simulink model "WMMSupportingForcesGP2020a"  (R2020a)
settings: Solver=ode23t  StartTime=0.0  StopTime=inf  FixedStep=.001  RelTol=1e-3  AbsTol=1e-3
InitFcn:
  | InitializeSimulationGP
  | SimulationParametersGP
values from neighbouring files (symbols this model uses):
  B11_r_B11C = [0.23805608; 0.13201777; 0]    [InitializeSimulationGP.m]
  B11_r_B11Tc1 = [L11; 0; 0]    [InitializeSimulationGP.m]
  B11_Rot_Tc1 = eye(3)    [InitializeSimulationGP.m]
  B11cI = [0.28426000 -0.06487287 0;         -0.06487287  0.54237481 0;                   0  0          0.67891020]    [InitializeSimulationGP.m]
  B12_r_B12C = [0.60504569; 0.27199376; 0.00002484]    [InitializeSimulationGP.m]
  B12_r_B12Tc2 = [L12;0;0]    [InitializeSimulationGP.m]
  B12_Rot_Tc2 = eye(3)    [InitializeSimulationGP.m]
  B12cI = [1.18803886 -2.36786418 0.00280315;          -2.36786418 6.31493281 0.00022322;           0.00280315 0.00022322 7.40915161]    [InitializeSimulationGP.m]
  B31_r_B31C = [0.35781210 0 0]    [InitializeSimulationGP.m]
  B31_Rot_B41 = eye(3)    [InitializeSimulationGP.m]
  B31cI = diag([0.03150902 0.90735702 0.90763033])    [InitializeSimulationGP.m]
  B32_r_B32C = [0.35781210 0 0]    [InitializeSimulationGP.m]
  B32_Rot_B42 = eye(3)    [InitializeSimulationGP.m]
  B32cI = diag([0.03150902 0.90735702 0.90763033])    [InitializeSimulationGP.m]
  B41_r_B41C = [0.55785997 0 0]    [InitializeSimulationGP.m]
  B41_r_B41Tc1 = [lc1;0;0]    [InitializeSimulationGP.m]
  B41cI = diag([0.00370720 0.55759812 0.55785997])    [InitializeSimulationGP.m]
  B42_r_B42C = [0.55785997 0 0]    [InitializeSimulationGP.m]
  B42_r_B42Tc2 = [lc2; 0; 0]    [InitializeSimulationGP.m]
  B42cI = diag([0.00370720 0.55759812 0.55785997])    [InitializeSimulationGP.m]
  B52_r_B52C = [0 0 0.56802906]    [InitializeSimulationGP.m]
  B52_r_B52P32 = [lc3; 0; 0]    [InitializeSimulationGP.m]
  B52_Rot_P32 = eye(3)    [InitializeSimulationGP.m]
  B52cI = diag([0.91789884, 0.91790043, 0.00091463])    [InitializeSimulationGP.m]
  Bc1_r_Bc1B11 = [L1; 0; 0]    [InitializeSimulationGP.m]
  Bc1_r_Bc1B31 = [0;0;0]    [InitializeSimulationGP.m]
  Bc1_r_Bc1C = [0.14178771; 0.16555780; 0]    [InitializeSimulationGP.m]
  Bc1_V = [0;0;0;0;0;0]    [InitializeSimulationGP.m]
  Bc1cI = [+5.892211080 +5.476111360 -0.000019630;          +5.476111360 +28.66965601 -0.000024550;          -0.000019630 -0.000024550 +29.78955950]    [InitializeSimulationGP.m]
  Bc2_r_Bc2B12 = [L2;0;0]    [InitializeSimulationGP.m]
  Bc2_r_Bc2B32 = [0;0;0]    [InitializeSimulationGP.m]
  Bc2_r_Bc2C = [0.54319901; 0.10543875; 0]    [InitializeSimulationGP.m]
  Bc2cI = [0.48071390 0.52924041 0;          0.52924041 5.80912352 0;              0      0          5.97255351]    [InitializeSimulationGP.m]
  BC_r_BCBM = [xCA; yCA; zCA]    [SimulationParametersGP.m]
  BC_Rot_BM = eye(3)    [SimulationParametersGP.m]
  BCI = diag([100 1200 1000])    [SimulationParametersGP.m]
  beta1 = atan2d(374.261,935)*pi/180    [InitializeSimulationGP.m]
  beta2 = atan2d(45.757,373.313)*pi/180    [InitializeSimulationGP.m]
  beta3 = atan2d(139.50,1132.19)*pi/180    [InitializeSimulationGP.m]
  beta4 = atan2d(88.061,296.198)*pi/180    [InitializeSimulationGP.m]
  betaGround = 1e6    (= 1000000)    [SimulationParametersGP.m]
  BFL = 0.05    [SimulationParametersGP.m]
  BFR = 0.05    [SimulationParametersGP.m]
  BM_r_BMBMp = [0;0;0]    [SimulationParametersGP.m]
  BM_Rot_BMp = [cos(gamma) -sin(gamma) 0; sin(gamma) cos(gamma) 0; 0 0 1]    [SimulationParametersGP.m]
  BMp_r_BMpBc1 = [0.185;0;0.205]    [InitializeSimulationGP.m]
  BMp_Rot_Bc1 = [cos(alpha1) -sin(alpha1)  0;                  0            0       -1;                sin(alpha1)  cos(alpha1)  0]    [InitializeSimulationGP.m]
  BRL = 0.05    [SimulationParametersGP.m]
  BRR = 0.05    [SimulationParametersGP.m]
  cc = 0.0    (= 0)    [SimulationParametersGP.m]
  D22F = [0;0;0;0;0;0]    [InitializeSimulationGP.m]
  dT = 0.01    [SimulationParametersGP.m]
  g0 = 9.8066    [SimulationParametersGP.m]
  ground_stiffness = 1e8    (= 100000000)    [SimulationParametersGP.m]
  l1 = 1.15-cc    (= 1.15)    [SimulationParametersGP.m]
  L1 = 1.0071227324212    (= 1.00712273242)    [InitializeSimulationGP.m]
  L11 = 0.37610632101293    (= 0.376106321013)    [InitializeSimulationGP.m]
  L12 = 0.30901132665325    (= 0.309011326653)    [InitializeSimulationGP.m]
  l2 = 1.15+cc    (= 1.15)    [SimulationParametersGP.m]
  L2 = 1.132185817991    (= 1.13218581799)    [InitializeSimulationGP.m]
  lc1 = 0.745    [InitializeSimulationGP.m]
  lc2 = 0.745    [InitializeSimulationGP.m]
  mB11 = 25.52660174    [InitializeSimulationGP.m]
  mB12 = 33.92850233    [InitializeSimulationGP.m]
  mB31 = 17.36281648    [InitializeSimulationGP.m]
  mB32 = 17.36281648    [InitializeSimulationGP.m]
  mB41 = 10.34519231    [InitializeSimulationGP.m]
  mB42 = 10.34519231    [InitializeSimulationGP.m]
  mB52 = 6.73059863    [InitializeSimulationGP.m]
  mBC = 2200    [SimulationParametersGP.m]
  mBc1 = 307.29601379    [InitializeSimulationGP.m]
  mBc2 = 54.58702836    [InitializeSimulationGP.m]
  mFL = 60    [SimulationParametersGP.m]
  mFR = 60    [SimulationParametersGP.m]
  mP22 = 9.26136143    [InitializeSimulationGP.m]
  mP32 = 570.18877059    [InitializeSimulationGP.m]
  mRR = 60    [SimulationParametersGP.m]
  mw = mFL    (= 60)    [SimulationParametersGP.m]
  P22_r_P22C = [0.62192523 0 0]    [InitializeSimulationGP.m]
  P22_Rot_B52 = eye(3)    [InitializeSimulationGP.m]
  P22cI = diag([0.00662754, 1.48387017, 1.48398069])    [InitializeSimulationGP.m]
  P32_r_P32C = [0.25466704; -0.13034397; -0.01302248]    [InitializeSimulationGP.m]
  P32_r_P32D22 = [0.40499744871392; -0.13130517281345; -0.013385243295654]    [InitializeSimulationGP.m]
  P32_Rot_D22 = [1 0 0;              0 0.9707729441837 0.23999977258512;              0 -0.23999977258512 0.9707729441837]    [InitializeSimulationGP.m]
  P32cI = [46.81220713 0.38607676 -0.00453819;          0.38607676 71.92201786 -1.14320993;          -0.00453819 -1.14320993 67.38128576]    [InitializeSimulationGP.m]
  R0FL = 0.35    [SimulationParametersGP.m]
  R0FR = 0.35    [SimulationParametersGP.m]
  R0RL = 0.35    [SimulationParametersGP.m]
  R0RR = 0.35    [SimulationParametersGP.m]
  Rw = R0FL    (= 0.35)    [SimulationParametersGP.m]
  Tc1_r_Tc1Bc2 = [0.098495302558553; 0.01838181329939; 0]    [InitializeSimulationGP.m]
  Tc1_Rot_Bc2 = [cos(alpha2) -sin(alpha2) 0;                sin(alpha2)  cos(alpha2) 0;                0            0           1]    [InitializeSimulationGP.m]
  Tc2_r_Tc2P22 = [-0.048858374920227;0.36587359346146;0.035276938723102]    [InitializeSimulationGP.m]
  Tc2_Rot_P22 = [0.95853460763586 -0.27664713597974  0.0683942111482;                0.28497614981675  0.93051946315663 -0.23004808784757;                0                 0.23999977258511  0.9707729441837]    [InitializeSimulationGP.m]
  Th1A = 10*pi/180    (= 0.174532925199)    [InitializeSimulationGP.m]
  Th1B = 20*pi/180    (= 0.349065850399)    [InitializeSimulationGP.m]
  Th1f = 1    [InitializeSimulationGP.m]
  Th2A = 15*pi/180    (= 0.261799387799)    [InitializeSimulationGP.m]
  Th2B = -70*pi/180    (= -1.2217304764)    [InitializeSimulationGP.m]
  Th2f = 2    [InitializeSimulationGP.m]
  w = wFL    (= 0.875)    [SimulationParametersGP.m]
  W_r_WBc1 = [0.185;0;0.205]    [InitializeSimulationGP.m]
  W_Rot_Bc1 = [cos(alpha1) -sin(alpha1)  0;                  0            0       -1;                sin(alpha1)  cos(alpha1)  0]    [InitializeSimulationGP.m]
  x10 = 0.83    [InitializeSimulationGP.m]
  x20 = 0.83    [InitializeSimulationGP.m]
  x3A = 0.2    [InitializeSimulationGP.m]
  x3B = 0.3    [InitializeSimulationGP.m]
  x3f = 1    [InitializeSimulationGP.m]
  xCA = 0.5    [SimulationParametersGP.m]
  xf = [1;0;0;0;0;0]    [InitializeSimulationGP.m]
  yCA = 0    [SimulationParametersGP.m]
  zC = 0.45    [SimulationParametersGP.m]
  zCA = .25    (= 0.25)    [SimulationParametersGP.m]
  ztau = [0;0;0;0;0;1]    [InitializeSimulationGP.m]
undefined symbols (not defined in the file or in its folder): alphaFL_meas, alphaFR_meas, alphaRL_meas, alphaRR_meas, B11_V, B11Ftot, B12_U_Tc2, B12_V, B12Ftot, B31_r_B31B41, B31_V, B31FTot, B32_r_B32B42, B32_U_B42, B32_V, B32FTot, B41_V, B41FTot, B42_Rot_Tc2, B42_U_Tc2, B42_V, B42FTot, B52_U_P32, B52_V, B52Ftot, Bc1Tot, Bc2_Rot_B12, Bc2_Rot_B32, Bc2_U_B12, Bc2_U_B32, Bc2_V, Bc2Tot, betaC_meas, D22_V, deltaFL_cmd, deltaFL_meas, deltaFR_cmd, deltaFR_meas, deltaRL_cmd, deltaRL_meas, deltaRR_cmd, deltaRR_meas, dOmegaFL_meas, dOmegaFR_meas, dOmegaRL_meas, dOmegaRR_meas, dPsi_meas, dq1, dq11, dq12, dq2, dq21, dq22, dx1, dx2, Floor, FTot_S1, FTot_S2P, FTot_S2R, FzFL ... (+63)
libraries: sm_lib x94, nesl_utility x63, simulink x5
(part 5 of 11)

== system WMMSupportingForcesGP2020a/Mobile Manipulator in Simscape/get_measurements ==
  MATLAB Function : MATLAB Function  TreatAsAtomicUnit=on
  PS-Simulink Converter{1..2,15..16} (4 alike) : nesl_utility/PS-Simulink Converter  PhysicalDomain=network_engine_domain  SubClassName=ps_output  LeftPortType=input  RightPortType=output  PseudoPeriodic=off  Frequencies=[]  Unit=inherit  AffineConversion=off
      settings: SourceProductBaseCode=PW,SS
  Rate Transition{,1..5} (6 alike) : RateTransition  OutPortSampleTime=dT
  Reshape : Reshape  OutputDimensionality=Customize  OutputDimensions=[3,3]
  measVCwrtW : sm_lib/Frames and Transforms/Transform Sensor  MeasurementFrame=NonRotatingFollower  SenseAngle=off  SenseAxis=off  SenseAngle1=off  SenseAngle2=off  SenseAngle3=off  SenseQ=off  SenseR=on  SenseOmegaX=off  SenseOmegaY=off  SenseOmegaZ=on  SenseOmega1=off  SenseOmega2=off  SenseOmega3=off  SenseQDot=off  SenseRDot=off  SenseAlphaX=off  SenseAlphaY=off  SenseAlphaZ=off  SenseAlpha1=off  SenseAlpha2=off  SenseAlpha3=off  SenseQDDot=off  SenseRDDot=off  SenseX=off  SenseY=off  SenseZ=off  SenseRad=off  SenseAzim=off  SenseDist=off  SenseInc=off  SenseXDot=on  SenseYDot=on  SenseZDot=off  SenseRadDot=off  SenseAzimDot=off  SenseDistDot=off  SenseIncDot=off  SenseXDDot=off  SenseYDDot=off  SenseZDDot=off  SenseRadDDot=off  SenseAzimDDot=off  SenseDistDDot=off  SenseIncDDot=off
  W : PMIOPort  Side=Left
  BC : PMIOPort  Port=2  Side=Left
  Theta_meas : Outport
  Phi_meas : Outport  Port=2
  Psi_meas : Outport  Port=3
  dPsi_meas : Outport  Port=4
  VCx_meas : Outport  Port=5
  VCy_meas : Outport  Port=6
  wires:
  PS-Simulink Converter15/1 -> Rate Transition/1
  PS-Simulink Converter1/1 -> Reshape/1
  Reshape/1 -> MATLAB Function/1(u)
  Rate Transition/1 -> dPsi_meas/1
  PS-Simulink Converter16/1 -> Rate Transition1/1
  Rate Transition1/1 -> VCx_meas/1
  PS-Simulink Converter2/1 -> Rate Transition2/1
  Rate Transition2/1 -> VCy_meas/1
  MATLAB Function/3(Psi) -> Rate Transition4/1
  MATLAB Function/2(Phi) -> Rate Transition3/1
  MATLAB Function/1(Theta) -> Rate Transition5/1
  Rate Transition4/1 -> Psi_meas/1
  Rate Transition3/1 -> Phi_meas/1
  Rate Transition5/1 -> Theta_meas/1
  connections:
  BC/RConn1 -- measVCwrtW/RConn1
  W/RConn1 -- measVCwrtW/LConn1
  measVCwrtW/RConn2 -- PS-Simulink Converter1/LConn1
  measVCwrtW/RConn5 -- PS-Simulink Converter2/LConn1
  measVCwrtW/RConn3 -- PS-Simulink Converter15/LConn1
  measVCwrtW/RConn4 -- PS-Simulink Converter16/LConn1

== system WMMSupportingForcesGP2020a/Mobile Manipulator in Simscape/meas_FLwheel_kinematic_quantities_in_Simscape ==
  Bus Creator : BusCreator  Inputs=alphaFL_meas,VFL_meas,VxFL_meas,dOmegaFL_meas,kappaFL_meas,ReFL
  Connection Label1 : ConnectionLabel  Label=W
  Connection Label2 : ConnectionLabel  Label=W
  Connection Label56 : ConnectionLabel  Label=W
  Constant : Constant  Value=R0FL
  PS-Simulink Converter1 : nesl_utility/PS-Simulink Converter  PhysicalDomain=network_engine_domain  SubClassName=ps_output  LeftPortType=input  RightPortType=output  PseudoPeriodic=off  Frequencies=[]  Unit=inherit  AffineConversion=off
      settings: SourceProductBaseCode=PW,SS
  PS-Simulink Converter2 : nesl_utility/PS-Simulink Converter  PhysicalDomain=network_engine_domain  SubClassName=ps_output  LeftPortType=input  RightPortType=output  PseudoPeriodic=off  Frequencies=[]  Unit=inherit  AffineConversion=off
      settings: SourceProductBaseCode=PW,SS
  PS-Simulink Converter4 : nesl_utility/PS-Simulink Converter  PhysicalDomain=network_engine_domain  SubClassName=ps_output  LeftPortType=input  RightPortType=output  PseudoPeriodic=off  Frequencies=[]  Unit=inherit  AffineConversion=off
      settings: SourceProductBaseCode=PW,SS
  calc_longitudinal_slip_FL : Subsystem
  meas_VFL : Subsystem
  meas_VFL1 : Subsystem
  meas_WFL_to_W_in_WFL : sm_lib/Frames and Transforms/Transform Sensor  MeasurementFrame=NonRotatingFollower  SenseAngle=off  SenseAxis=off  SenseAngle1=off  SenseAngle2=off  SenseAngle3=off  SenseQ=off  SenseR=off  SenseOmegaX=off  SenseOmegaY=off  SenseOmegaZ=off  SenseOmega1=off  SenseOmega2=off  SenseOmega3=off  SenseQDot=off  SenseRDot=off  SenseAlphaX=off  SenseAlphaY=off  SenseAlphaZ=off  SenseAlpha1=off  SenseAlpha2=off  SenseAlpha3=off  SenseQDDot=off  SenseRDDot=off  SenseX=off  SenseY=off  SenseZ=off  SenseRad=off  SenseAzim=off  SenseDist=off  SenseInc=off  SenseXDot=on  SenseYDot=on  SenseZDot=off  SenseRadDot=off  SenseAzimDot=off  SenseDistDot=off  SenseIncDot=off  SenseXDDot=off  SenseYDDot=off  SenseZDDot=off  SenseRadDDot=off  SenseAzimDDot=off  SenseDistDDot=off  SenseIncDDot=off
  meas_WFLp_to_W_in_WFLp : sm_lib/Frames and Transforms/Transform Sensor  MeasurementFrame=NonRotatingFollower  SenseAngle=off  SenseAxis=off  SenseAngle1=off  SenseAngle2=off  SenseAngle3=off  SenseQ=off  SenseR=off  SenseOmegaX=off  SenseOmegaY=on  SenseOmegaZ=off  SenseOmega1=off  SenseOmega2=off  SenseOmega3=off  SenseQDot=off  SenseRDot=off  SenseAlphaX=off  SenseAlphaY=off  SenseAlphaZ=off  SenseAlpha1=off  SenseAlpha2=off  SenseAlpha3=off  SenseQDDot=off  SenseRDDot=off  SenseX=off  SenseY=off  SenseZ=off  SenseRad=off  SenseAzim=off  SenseDist=off  SenseInc=off  SenseXDot=off  SenseYDot=off  SenseZDot=off  SenseRadDot=off  SenseAzimDot=off  SenseDistDot=off  SenseIncDot=off  SenseXDDot=off  SenseYDDot=off  SenseZDDot=off  SenseRadDDot=off  SenseAzimDDot=off  SenseDistDDot=off  SenseIncDDot=off
  W : PMIOPort  Side=Left
  WFL : PMIOPort  Port=2  Side=Left
  WFLp : PMIOPort  Port=3  Side=Left
  FL_kin : Outport
  wires:
  [kappaFL_meas] -> Bus Creator/5  "kappaFL_meas"
  [dOmegaFL_meas] -> Bus Creator/4  "dOmegaFL_meas"
  [VxFL_meas] -> calc_longitudinal_slip_FL/3(VxFL_meas)
  [ReFL] -> calc_longitudinal_slip_FL/2(ReFL)
  Constant/1 -> [ReFL]
  [dOmegaFL_meas] -> calc_longitudinal_slip_FL/1(dOmegaFL_meas)
  calc_longitudinal_slip_FL/1(kappaFL_meas) -> [kappaFL_meas]
  PS-Simulink Converter1/1 -> [dOmegaFL_meas]
  [VxFL_meas] -> meas_VFL/1(VFLx_meas)
  [VyFL_meas] -> meas_VFL/2(VFLy_meas)
  PS-Simulink Converter2/1 -> [VxFL_meas]
  PS-Simulink Converter4/1 -> [VyFL_meas]
  [alphaFL_meas] -> Bus Creator/1  "alphaFL_meas"
  meas_VFL/1(VFL_meas) -> [VFL_meas]
  [VFL_meas] -> Bus Creator/2  "VFL_meas"
  [VxFL_meas] -> Bus Creator/3  "VxFL_meas"
  Bus Creator/1 -> [FL_kin]
  [ReFL] -> Bus Creator/6  "ReFL"
  [FL_kin] -> FL_kin/1
  [VyFL_meas] -> meas_VFL1/2(VFLy_meas)
  [VxFL_meas] -> meas_VFL1/1(VFLx_meas)
  meas_VFL1/1(alphaFL_meas) -> [alphaFL_meas]
  connections:
  meas_WFLp_to_W_in_WFLp/RConn1 -- WFLp/RConn1
  Connection Label1/LConn1 -- meas_WFL_to_W_in_WFL/LConn1
  Connection Label56/LConn1 -- W/RConn1
  PS-Simulink Converter1/LConn1 -- meas_WFLp_to_W_in_WFLp/RConn2
  Connection Label2/LConn1 -- meas_WFLp_to_W_in_WFLp/LConn1
  meas_WFL_to_W_in_WFL/RConn3 -- PS-Simulink Converter4/LConn1
  PS-Simulink Converter2/LConn1 -- meas_WFL_to_W_in_WFL/RConn2
  meas_WFL_to_W_in_WFL/RConn1 -- WFL/RConn1

== system WMMSupportingForcesGP2020a/Mobile Manipulator in Simscape/meas_FRwheel_kinematic_quantities_in_Simscape ==
  Bus Creator : BusCreator  Inputs=alphaFR_meas,VFR_meas,VxFR_meas,dOmegaFR_meas,kappaFR_meas,ReFR
  Connection Label1 : ConnectionLabel  Label=W
  Connection Label2 : ConnectionLabel  Label=W
  Connection Label56 : ConnectionLabel  Label=W
  Constant : Constant  Value=R0FR
  PS-Simulink Converter1 : nesl_utility/PS-Simulink Converter  PhysicalDomain=network_engine_domain  SubClassName=ps_output  LeftPortType=input  RightPortType=output  PseudoPeriodic=off  Frequencies=[]  Unit=inherit  AffineConversion=off
      settings: SourceProductBaseCode=PW,SS
  PS-Simulink Converter2 : nesl_utility/PS-Simulink Converter  PhysicalDomain=network_engine_domain  SubClassName=ps_output  LeftPortType=input  RightPortType=output  PseudoPeriodic=off  Frequencies=[]  Unit=inherit  AffineConversion=off
      settings: SourceProductBaseCode=PW,SS
  PS-Simulink Converter4 : nesl_utility/PS-Simulink Converter  PhysicalDomain=network_engine_domain  SubClassName=ps_output  LeftPortType=input  RightPortType=output  PseudoPeriodic=off  Frequencies=[]  Unit=inherit  AffineConversion=off
      settings: SourceProductBaseCode=PW,SS
  calc_longitudinal_slip_FR : Subsystem
  meas_VFL1 : Subsystem
  meas_VFR : Subsystem
  meas_WFR_to_W_in_WFR : sm_lib/Frames and Transforms/Transform Sensor  MeasurementFrame=NonRotatingFollower  SenseAngle=off  SenseAxis=off  SenseAngle1=off  SenseAngle2=off  SenseAngle3=off  SenseQ=off  SenseR=off  SenseOmegaX=off  SenseOmegaY=off  SenseOmegaZ=off  SenseOmega1=off  SenseOmega2=off  SenseOmega3=off  SenseQDot=off  SenseRDot=off  SenseAlphaX=off  SenseAlphaY=off  SenseAlphaZ=off  SenseAlpha1=off  SenseAlpha2=off  SenseAlpha3=off  SenseQDDot=off  SenseRDDot=off  SenseX=off  SenseY=off  SenseZ=off  SenseRad=off  SenseAzim=off  SenseDist=off  SenseInc=off  SenseXDot=on  SenseYDot=on  SenseZDot=off  SenseRadDot=off  SenseAzimDot=off  SenseDistDot=off  SenseIncDot=off  SenseXDDot=off  SenseYDDot=off  SenseZDDot=off  SenseRadDDot=off  SenseAzimDDot=off  SenseDistDDot=off  SenseIncDDot=off
  meas_WFRp_to_W_in_WFRp : sm_lib/Frames and Transforms/Transform Sensor  MeasurementFrame=NonRotatingFollower  SenseAngle=off  SenseAxis=off  SenseAngle1=off  SenseAngle2=off  SenseAngle3=off  SenseQ=off  SenseR=off  SenseOmegaX=off  SenseOmegaY=on  SenseOmegaZ=off  SenseOmega1=off  SenseOmega2=off  SenseOmega3=off  SenseQDot=off  SenseRDot=off  SenseAlphaX=off  SenseAlphaY=off  SenseAlphaZ=off  SenseAlpha1=off  SenseAlpha2=off  SenseAlpha3=off  SenseQDDot=off  SenseRDDot=off  SenseX=off  SenseY=off  SenseZ=off  SenseRad=off  SenseAzim=off  SenseDist=off  SenseInc=off  SenseXDot=off  SenseYDot=off  SenseZDot=off  SenseRadDot=off  SenseAzimDot=off  SenseDistDot=off  SenseIncDot=off  SenseXDDot=off  SenseYDDot=off  SenseZDDot=off  SenseRadDDot=off  SenseAzimDDot=off  SenseDistDDot=off  SenseIncDDot=off
  W : PMIOPort  Side=Left
  WFR : PMIOPort  Port=2  Side=Left
  WFRp : PMIOPort  Port=3  Side=Left
  FR_kin : Outport
  wires:
  meas_VFR/1(VFR_meas) -> [VFR_meas]
  PS-Simulink Converter4/1 -> [VyFR_meas]
  PS-Simulink Converter2/1 -> [VxFR_meas]
  [VyFR_meas] -> meas_VFR/2(VFRy_meas)
  [VxFR_meas] -> meas_VFR/1(VFRx_meas)
  PS-Simulink Converter1/1 -> [dOmegaFR_meas]
  calc_longitudinal_slip_FR/1(kappaFR_meas) -> [kappaFR_meas]
  [dOmegaFR_meas] -> calc_longitudinal_slip_FR/1(dOmegaFR_meas)
  Constant/1 -> [ReFR]
  [ReFR] -> calc_longitudinal_slip_FR/2(ReFR)
  [VxFR_meas] -> calc_longitudinal_slip_FR/3(VxFR_meas)
  [dOmegaFR_meas] -> Bus Creator/4  "dOmegaFR_meas"
  [VxFR_meas] -> Bus Creator/3  "VxFR_meas"
  [alphaFR_meas] -> Bus Creator/1  "alphaFR_meas"
  [VFR_meas] -> Bus Creator/2  "VFR_meas"
  [kappaFR_meas] -> Bus Creator/5  "kappaFR_meas"
  Bus Creator/1 -> [FR_kin]
  [FR_kin] -> FR_kin/1
  [ReFR] -> Bus Creator/6  "ReFR"
  [VxFR_meas] -> meas_VFL1/1(VFRx_meas)
  [VyFR_meas] -> meas_VFL1/2(VFRy_meas)
  meas_VFL1/1(alphaFR_meas) -> [alphaFR_meas]
  connections:
  meas_WFR_to_W_in_WFR/RConn1 -- WFR/RConn1
  PS-Simulink Converter2/LConn1 -- meas_WFR_to_W_in_WFR/RConn2
  meas_WFR_to_W_in_WFR/RConn3 -- PS-Simulink Converter4/LConn1
  Connection Label2/LConn1 -- meas_WFRp_to_W_in_WFRp/LConn1
  PS-Simulink Converter1/LConn1 -- meas_WFRp_to_W_in_WFRp/RConn2
  Connection Label56/LConn1 -- W/RConn1
  Connection Label1/LConn1 -- meas_WFR_to_W_in_WFR/LConn1
  meas_WFRp_to_W_in_WFRp/RConn1 -- WFRp/RConn1

== system WMMSupportingForcesGP2020a/Mobile Manipulator in Simscape/meas_RLwheel_kinematic_quantities_in_Simscape ==
  Bus Creator : BusCreator  Inputs=alphaRL_meas,VRL_meas,VxRL_meas,dOmegaRL_meas,kappaRL_meas,ReRL
  Connection Label1 : ConnectionLabel  Label=W
  Connection Label2 : ConnectionLabel  Label=W
  Connection Label56 : ConnectionLabel  Label=W
  Constant : Constant  Value=R0RL
  PS-Simulink Converter1 : nesl_utility/PS-Simulink Converter  PhysicalDomain=network_engine_domain  SubClassName=ps_output  LeftPortType=input  RightPortType=output  PseudoPeriodic=off  Frequencies=[]  Unit=inherit  AffineConversion=off
      settings: SourceProductBaseCode=PW,SS
  PS-Simulink Converter2 : nesl_utility/PS-Simulink Converter  PhysicalDomain=network_engine_domain  SubClassName=ps_output  LeftPortType=input  RightPortType=output  PseudoPeriodic=off  Frequencies=[]  Unit=inherit  AffineConversion=off
      settings: SourceProductBaseCode=PW,SS
  PS-Simulink Converter4 : nesl_utility/PS-Simulink Converter  PhysicalDomain=network_engine_domain  SubClassName=ps_output  LeftPortType=input  RightPortType=output  PseudoPeriodic=off  Frequencies=[]  Unit=inherit  AffineConversion=off
      settings: SourceProductBaseCode=PW,SS
  calc_longitudinal_slip_RL : Subsystem
  meas_VFL1 : Subsystem
  meas_VRL : Subsystem
  meas_WRL_to_W_in_WRL : sm_lib/Frames and Transforms/Transform Sensor  MeasurementFrame=NonRotatingFollower  SenseAngle=off  SenseAxis=off  SenseAngle1=off  SenseAngle2=off  SenseAngle3=off  SenseQ=off  SenseR=off  SenseOmegaX=off  SenseOmegaY=off  SenseOmegaZ=off  SenseOmega1=off  SenseOmega2=off  SenseOmega3=off  SenseQDot=off  SenseRDot=off  SenseAlphaX=off  SenseAlphaY=off  SenseAlphaZ=off  SenseAlpha1=off  SenseAlpha2=off  SenseAlpha3=off  SenseQDDot=off  SenseRDDot=off  SenseX=off  SenseY=off  SenseZ=off  SenseRad=off  SenseAzim=off  SenseDist=off  SenseInc=off  SenseXDot=on  SenseYDot=on  SenseZDot=off  SenseRadDot=off  SenseAzimDot=off  SenseDistDot=off  SenseIncDot=off  SenseXDDot=off  SenseYDDot=off  SenseZDDot=off  SenseRadDDot=off  SenseAzimDDot=off  SenseDistDDot=off  SenseIncDDot=off
  meas_WRLp_to_W_in_WRLp : sm_lib/Frames and Transforms/Transform Sensor  MeasurementFrame=NonRotatingFollower  SenseAngle=off  SenseAxis=off  SenseAngle1=off  SenseAngle2=off  SenseAngle3=off  SenseQ=off  SenseR=off  SenseOmegaX=off  SenseOmegaY=on  SenseOmegaZ=off  SenseOmega1=off  SenseOmega2=off  SenseOmega3=off  SenseQDot=off  SenseRDot=off  SenseAlphaX=off  SenseAlphaY=off  SenseAlphaZ=off  SenseAlpha1=off  SenseAlpha2=off  SenseAlpha3=off  SenseQDDot=off  SenseRDDot=off  SenseX=off  SenseY=off  SenseZ=off  SenseRad=off  SenseAzim=off  SenseDist=off  SenseInc=off  SenseXDot=off  SenseYDot=off  SenseZDot=off  SenseRadDot=off  SenseAzimDot=off  SenseDistDot=off  SenseIncDot=off  SenseXDDot=off  SenseYDDot=off  SenseZDDot=off  SenseRadDDot=off  SenseAzimDDot=off  SenseDistDDot=off  SenseIncDDot=off
  W : PMIOPort  Side=Left
  WRL : PMIOPort  Port=2  Side=Left
  WRLp : PMIOPort  Port=3  Side=Left
  RL_kin : Outport
  wires:
  meas_VRL/1(VRL_meas) -> [VRL_meas]
  PS-Simulink Converter4/1 -> [VyRL_meas]
  PS-Simulink Converter2/1 -> [VxRL_meas]
  [VyRL_meas] -> meas_VRL/2(VRLy_meas)
  [VxRL_meas] -> meas_VRL/1(VRLx_meas)
  PS-Simulink Converter1/1 -> [dOmegaRL_meas]
  calc_longitudinal_slip_RL/1(kappaRL_meas) -> [kappaRL_meas]
  [dOmegaRL_meas] -> calc_longitudinal_slip_RL/1(dOmegaRL_meas)
  Constant/1 -> [ReRL]
  [ReRL] -> calc_longitudinal_slip_RL/2(ReRL)
  [VxRL_meas] -> calc_longitudinal_slip_RL/3(VxRL_meas)
  [dOmegaRL_meas] -> Bus Creator/4  "dOmegaRL_meas"
  [VxRL_meas] -> Bus Creator/3  "VxRL_meas"
  [alphaRL_meas] -> Bus Creator/1  "alphaRL_meas"
  [VRL_meas] -> Bus Creator/2  "VRL_meas"
  [kappaRL_meas] -> Bus Creator/5  "kappaRL_meas"
  Bus Creator/1 -> [RL_kin]
  [RL_kin] -> RL_kin/1
  [ReRL] -> Bus Creator/6  "ReRL"
  [VxRL_meas] -> meas_VFL1/1(VRLx_meas)
  [VyRL_meas] -> meas_VFL1/2(VRLy_meas)
  meas_VFL1/1(alphaRL_meas) -> [alphaRL_meas]
  connections:
  meas_WRL_to_W_in_WRL/RConn1 -- WRL/RConn1
  PS-Simulink Converter2/LConn1 -- meas_WRL_to_W_in_WRL/RConn2
  meas_WRL_to_W_in_WRL/RConn3 -- PS-Simulink Converter4/LConn1
  Connection Label2/LConn1 -- meas_WRLp_to_W_in_WRLp/LConn1
  PS-Simulink Converter1/LConn1 -- meas_WRLp_to_W_in_WRLp/RConn2
  Connection Label56/LConn1 -- W/RConn1
  Connection Label1/LConn1 -- meas_WRL_to_W_in_WRL/LConn1
  meas_WRLp_to_W_in_WRLp/RConn1 -- WRLp/RConn1

== system WMMSupportingForcesGP2020a/Mobile Manipulator in Simscape/meas_RRwheel_kinematic_quantities_in_Simscape ==
  Bus Creator : BusCreator  Inputs=alphaRR_meas,VRR_meas,VxRR_meas,dOmegaRR_meas,kappaRR_meas,ReRR
  Connection Label1 : ConnectionLabel  Label=W
  Connection Label2 : ConnectionLabel  Label=W
  Connection Label56 : ConnectionLabel  Label=W
  Constant : Constant  Value=R0RR
  PS-Simulink Converter1 : nesl_utility/PS-Simulink Converter  PhysicalDomain=network_engine_domain  SubClassName=ps_output  LeftPortType=input  RightPortType=output  PseudoPeriodic=off  Frequencies=[]  Unit=inherit  AffineConversion=off
      settings: SourceProductBaseCode=PW,SS
  PS-Simulink Converter2 : nesl_utility/PS-Simulink Converter  PhysicalDomain=network_engine_domain  SubClassName=ps_output  LeftPortType=input  RightPortType=output  PseudoPeriodic=off  Frequencies=[]  Unit=inherit  AffineConversion=off
      settings: SourceProductBaseCode=PW,SS
  PS-Simulink Converter4 : nesl_utility/PS-Simulink Converter  PhysicalDomain=network_engine_domain  SubClassName=ps_output  LeftPortType=input  RightPortType=output  PseudoPeriodic=off  Frequencies=[]  Unit=inherit  AffineConversion=off
      settings: SourceProductBaseCode=PW,SS
  calc_longitudinal_slip_RR : Subsystem
  meas_VFL1 : Subsystem
  meas_VRR : Subsystem
  meas_WRR_to_W_in_WRR : sm_lib/Frames and Transforms/Transform Sensor  MeasurementFrame=NonRotatingFollower  SenseAngle=off  SenseAxis=off  SenseAngle1=off  SenseAngle2=off  SenseAngle3=off  SenseQ=off  SenseR=off  SenseOmegaX=off  SenseOmegaY=off  SenseOmegaZ=off  SenseOmega1=off  SenseOmega2=off  SenseOmega3=off  SenseQDot=off  SenseRDot=off  SenseAlphaX=off  SenseAlphaY=off  SenseAlphaZ=off  SenseAlpha1=off  SenseAlpha2=off  SenseAlpha3=off  SenseQDDot=off  SenseRDDot=off  SenseX=off  SenseY=off  SenseZ=off  SenseRad=off  SenseAzim=off  SenseDist=off  SenseInc=off  SenseXDot=on  SenseYDot=on  SenseZDot=off  SenseRadDot=off  SenseAzimDot=off  SenseDistDot=off  SenseIncDot=off  SenseXDDot=off  SenseYDDot=off  SenseZDDot=off  SenseRadDDot=off  SenseAzimDDot=off  SenseDistDDot=off  SenseIncDDot=off
  meas_WRRp_to_W_in_WRRp : sm_lib/Frames and Transforms/Transform Sensor  MeasurementFrame=NonRotatingFollower  SenseAngle=off  SenseAxis=off  SenseAngle1=off  SenseAngle2=off  SenseAngle3=off  SenseQ=off  SenseR=off  SenseOmegaX=off  SenseOmegaY=on  SenseOmegaZ=off  SenseOmega1=off  SenseOmega2=off  SenseOmega3=off  SenseQDot=off  SenseRDot=off  SenseAlphaX=off  SenseAlphaY=off  SenseAlphaZ=off  SenseAlpha1=off  SenseAlpha2=off  SenseAlpha3=off  SenseQDDot=off  SenseRDDot=off  SenseX=off  SenseY=off  SenseZ=off  SenseRad=off  SenseAzim=off  SenseDist=off  SenseInc=off  SenseXDot=off  SenseYDot=off  SenseZDot=off  SenseRadDot=off  SenseAzimDot=off  SenseDistDot=off  SenseIncDot=off  SenseXDDot=off  SenseYDDot=off  SenseZDDot=off  SenseRadDDot=off  SenseAzimDDot=off  SenseDistDDot=off  SenseIncDDot=off
  W : PMIOPort  Side=Left
  WRR : PMIOPort  Port=2  Side=Left
  WRRp : PMIOPort  Port=3  Side=Left
  RR_kin : Outport
  wires:
  [VxRR_meas] -> calc_longitudinal_slip_RR/3(VxRR_meas)
  [ReRR] -> calc_longitudinal_slip_RR/2(ReRR)
  Constant/1 -> [ReRR]
  [dOmegaRR_meas] -> calc_longitudinal_slip_RR/1(dOmegaRR_meas)
  calc_longitudinal_slip_RR/1(kappaRR_meas) -> [kappaRR_meas]
  PS-Simulink Converter1/1 -> [dOmegaRR_meas]
  [VxRR_meas] -> meas_VRR/1(VRRx_meas)
  [VyRR_meas] -> meas_VRR/2(VRRy_meas)
  PS-Simulink Converter2/1 -> [VxRR_meas]
  PS-Simulink Converter4/1 -> [VyRR_meas]
  meas_VRR/1(VRR_meas) -> [VRR_meas]
  [RR_kin] -> RR_kin/1
  [kappaRR_meas] -> Bus Creator/5  "kappaRR_meas"
  [ReRR] -> Bus Creator/6  "ReRR"
  Bus Creator/1 -> [RR_kin]
  [alphaRR_meas] -> Bus Creator/1  "alphaRR_meas"
  [VRR_meas] -> Bus Creator/2  "VRR_meas"
  [dOmegaRR_meas] -> Bus Creator/4  "dOmegaRR_meas"
  [VxRR_meas] -> Bus Creator/3  "VxRR_meas"
  [VxRR_meas] -> meas_VFL1/1(VRRx_meas)
  [VyRR_meas] -> meas_VFL1/2(VRRy_meas)
  meas_VFL1/1(alphaRR_meas) -> [alphaRR_meas]
  connections:
  meas_WRRp_to_W_in_WRRp/RConn1 -- WRRp/RConn1
  Connection Label1/LConn1 -- meas_WRR_to_W_in_WRR/LConn1
  Connection Label56/LConn1 -- W/RConn1
  PS-Simulink Converter1/LConn1 -- meas_WRRp_to_W_in_WRRp/RConn2
  Connection Label2/LConn1 -- meas_WRRp_to_W_in_WRRp/LConn1
  meas_WRR_to_W_in_WRR/RConn3 -- PS-Simulink Converter4/LConn1
  PS-Simulink Converter2/LConn1 -- meas_WRR_to_W_in_WRR/RConn2
  meas_WRR_to_W_in_WRR/RConn1 -- WRR/RConn1

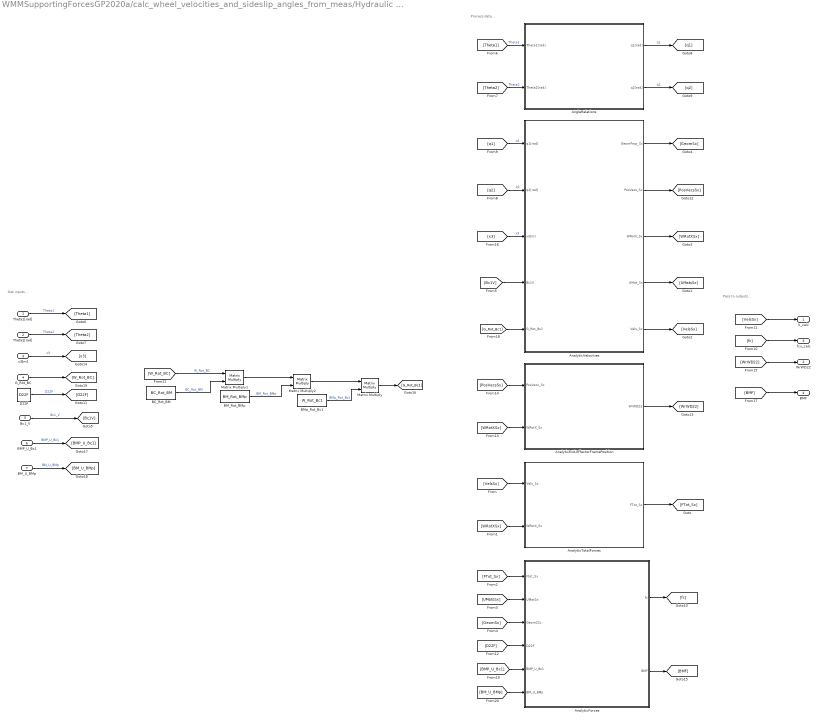
== system WMMSupportingForcesGP2020a/calc_wheel_velocities_and_sideslip_angles_from_meas/Hydraulic manipulator, calculation ==
  note: Pass to outputs...
  note: Get inputs...
  note: Process data...
  Theta1[rad] : Inport
  Theta2[rad] : Inport  Port=2
  x3[m] : Inport  Port=3
  G_Rot_BC : Inport  Port=4
  Bc1_V : Inport  Port=5
  BMP_U_Bc1 : Inport  Port=6
  BM_U_BMp : Inport  Port=7
  AnalyticEnd-EffectorFramePosition : Subsystem
  AnalyticForces : Subsystem
  AnalyticTotalForces : Subsystem
  AnalyticVelocities : Subsystem
  AngleRelations : Subsystem
  BC_Rot_BM : Constant  Value=BC_Rot_BM
  BM_Rot_BMp : Constant  Value=BM_Rot_BMp
  BMp_Rot_Bc1 : Constant  Value=W_Rot_Bc1
  D22F : Constant  Value=D22F
  Matrix Multiply : Product  Multiplication=Matrix(*)
  Matrix Multiply1 : Product  Multiplication=Matrix(*)
  Matrix Multiply2 : Product  Multiplication=Matrix(*)
  V_calc : Outport
  WrWD22 : Outport  Port=2
  fcx_calc : Outport  Port=3
  BMF : Outport  Port=4
  wires:
  AnalyticTotalForces/1(FTot_Sx) -> [FTot_Sx]
  AnalyticVelocities/1(GeomProp_Sx) -> [GeomSx]
  AnalyticVelocities/4(UMat_Sx) -> [UMatsSx]
  [UMatsSx] -> AnalyticForces/2(UMatSx)
  [VelsSx] -> AnalyticTotalForces/1(Vels_Sx)
  [GeomSx] -> AnalyticForces/3(GeomCCx)
  AnalyticVelocities/3(WRotX_Sx) -> [WRotXSx]
  [WRotXSx] -> AnalyticTotalForces/2(WRotX_Sx)
  [FTot_Sx] -> AnalyticForces/1(Ftot_Sx)
  AnalyticVelocities/5(Vels_Sx) -> [VelsSx]
  Theta1[rad]/1 -> [Theta1]  "Theta1"
  Theta2[rad]/1 -> [Theta2]  "Theta2"
  [Theta1] -> AngleRelations/1(Theta1[rad])  "Theta1"
  [Theta2] -> AngleRelations/2(Theta2[rad])  "Theta2"
  AngleRelations/1(q1[rad]) -> [q1]  "q1"
  AngleRelations/2(q2[rad]) -> [q2]  "q2"
  [q2] -> AnalyticVelocities/2(q2[rad])  "q2"
  [q1] -> AnalyticVelocities/1(q1[rad])  "q1"
  AnalyticForces/1(fc) -> [fc]
  [fc] -> fcx_calc/1
  [VelsSx] -> V_calc/1
  [D22F] -> AnalyticForces/4(D22F)
  [WRotXSx] -> AnalyticEnd-EffectorFramePosition/2(WRotX_Sx)
  AnalyticVelocities/2(PosVecs_Sx) -> [PosVecsSx]
  [PosVecsSx] -> AnalyticEnd-EffectorFramePosition/1(PosVecs_Sx)
  AnalyticEnd-EffectorFramePosition/1(WrWD22) -> [WrWD22]
  [WrWD22] -> WrWD22/1
  D22F/1 -> [D22F]  "D22F"
  x3[m]/1 -> [x3]  "x3"
  [x3] -> AnalyticVelocities/3(x3[m])  "x3"
  Bc1_V/1 -> [Bc1V]  "Bc1_V"
  [Bc1V] -> AnalyticVelocities/4(Bc1V)
  AnalyticForces/2(BMF) -> [BMF]
  [BMF] -> BMF/1
  [G_Rot_Bc1] -> AnalyticVelocities/5(G_Rot_Bc1)
  G_Rot_BC/1 -> [W_Rot_BC]
  BMP_U_Bc1/1 -> [BMP_U_Bc1]  "BMP_U_Bc1"
  [BMP_U_Bc1] -> AnalyticForces/5(BMP_U_Bc1)
  BM_U_BMp/1 -> [BM_U_BMp]  "BM_U_BMp"
  [BM_U_BMp] -> AnalyticForces/6(BM_U_BMp)
  Matrix Multiply1/1 -> Matrix Multiply2/1
  BMp_Rot_Bc1/1 -> Matrix Multiply/2  "BMp_Rot_Bc1"
  Matrix Multiply2/1 -> Matrix Multiply/1
  BC_Rot_BM/1 -> Matrix Multiply1/2  "BC_Rot_BM"
  BM_Rot_BMp/1 -> Matrix Multiply2/2  "BM_Rot_BMp"
  [W_Rot_BC] -> Matrix Multiply1/1  "W_Rot_BC"
  Matrix Multiply/1 -> [G_Rot_Bc1]

== system WMMSupportingForcesGP2020a/Mobile Manipulator in Simscape/GroundReactionFL/verticalForceFL ==
  hFL : Inport
  vzFL : Inport  Port=2
  Constant1 : Constant  Value=R0FL
  Subtract : Sum  Inputs=+-
  Sum1 : Sum  Inputs=|+-
  Tire Vertical Stiffness : Lookup_n-D  NumberOfTableDimensions=1  BreakpointsForDimension1=[-1 0 0.1]  Table=[ground_stiffness 0 0]  InternalRulePriority=Speed  RndMeth=Simplest  InputSameDT=on
  dampingForceFL : Subsystem
  FvertFL : Outport  VectorParamsAs1DForOutWhenUnconnected=off
  wires:
  Tire Vertical Stiffness/1 -> Sum1/1, dampingForceFL/1(Fz k)
  Subtract/1 -> Tire Vertical Stiffness/1
  Constant1/1 -> Subtract/2
  dampingForceFL/1(Fz d) -> Sum1/2
  vzFL/1 -> dampingForceFL/2(vz)
  Sum1/1 -> FvertFL/1
  hFL/1 -> Subtract/1

== system WMMSupportingForcesGP2020a/Mobile Manipulator in Simscape/GroundReactionFR/verticalForceFR ==
  hFR : Inport
  vzFR : Inport  Port=2
  Constant1 : Constant  Value=R0FR
  Subtract : Sum  Inputs=+-
  Sum1 : Sum  Inputs=|+-
  Tire Vertical Stiffness : Lookup_n-D  NumberOfTableDimensions=1  BreakpointsForDimension1=[-1 0 0.1]  Table=[ground_stiffness 0 0]  InternalRulePriority=Speed  RndMeth=Simplest  InputSameDT=on
  dampingForceFR : Subsystem
  FvertFR : Outport  VectorParamsAs1DForOutWhenUnconnected=off
  wires:
  Tire Vertical Stiffness/1 -> Sum1/1, dampingForceFR/1(Fz k)
  Subtract/1 -> Tire Vertical Stiffness/1
  Constant1/1 -> Subtract/2
  dampingForceFR/1(Fz d) -> Sum1/2
  vzFR/1 -> dampingForceFR/2(vz)
  Sum1/1 -> FvertFR/1
  hFR/1 -> Subtract/1

== system WMMSupportingForcesGP2020a/Mobile Manipulator in Simscape/GroundReactionRL/verticalForceRL ==
  hRL : Inport
  vzRL : Inport  Port=2
  Constant1 : Constant  Value=R0RL
  Subtract : Sum  Inputs=+-
  Sum1 : Sum  Inputs=|+-
  Tire Vertical Stiffness : Lookup_n-D  NumberOfTableDimensions=1  BreakpointsForDimension1=[-1 0 0.1]  Table=[ground_stiffness 0 0]  InternalRulePriority=Speed  RndMeth=Simplest  InputSameDT=on
  dampingForceRL : Subsystem
  FvertRL : Outport  VectorParamsAs1DForOutWhenUnconnected=off
  wires:
  Tire Vertical Stiffness/1 -> Sum1/1, dampingForceRL/1(Fz k)
  Subtract/1 -> Tire Vertical Stiffness/1
  Constant1/1 -> Subtract/2
  dampingForceRL/1(Fz d) -> Sum1/2
  vzRL/1 -> dampingForceRL/2(vz)
  Sum1/1 -> FvertRL/1
  hRL/1 -> Subtract/1

== system WMMSupportingForcesGP2020a/Mobile Manipulator in Simscape/GroundReactionRR/verticalForceRR ==
  hRR : Inport
  vzRR : Inport  Port=2
  Constant1 : Constant  Value=R0RR
  Subtract : Sum  Inputs=+-
  Sum1 : Sum  Inputs=|+-
  Tire Vertical Stiffness : Lookup_n-D  NumberOfTableDimensions=1  BreakpointsForDimension1=[-1 0 0.1]  Table=[ground_stiffness 0 0]  InternalRulePriority=Speed  RndMeth=Simplest  InputSameDT=on
  dampingForceRR : Subsystem
  FvertRR : Outport  VectorParamsAs1DForOutWhenUnconnected=off
  wires:
  Tire Vertical Stiffness/1 -> Sum1/1, dampingForceRR/1(Fz k)
  Subtract/1 -> Tire Vertical Stiffness/1
  Constant1/1 -> Subtract/2
  dampingForceRR/1(Fz d) -> Sum1/2
  vzRR/1 -> dampingForceRR/2(vz)
  Sum1/1 -> FvertRR/1
  hRR/1 -> Subtract/1

== system WMMSupportingForcesGP2020a/Mobile Manipulator in Simscape/Hydraulic manipulator, Simscape/Base ==
  note: Analytic derivatives
  Theta1[rad] : Inport
  BaseSolid : sm_lib/Body Elements/File Solid  ExtGeomFileName=01_BaseGP.STEP  UnitType=FromFile  ExtGeomFileUnits=m  StepReaderType=OCC  ExportConvexHullGeometry=off  InertiaType=Custom  Mass=307.29601379  MassUnits=kg  CenterOfMass=[0 -0.01488967 0.02139206]  CenterOfMassUnits=m  MomentsOfInertia=[29.78955950 5.25917100 29.30269608]  MomentsOfInertiaUnits=kg*m^2  ProductsOfInertia=[-3.89461427 -0.00003008 -0.00000910]  ProductsOfInertiaUnits=kg*m^2  BasedOnType=Density  Density=7300  DensityUnits=kg/m^3  DoExposeReferenceFrame=off  SerializedFrames=<Frames><Frame><Id>Frame1</Id><Value><Name>F2</Name><Origin><Source>GeometricFeature</Source><FeatureName>cylindrical surface 2</FeatureName></Origin><PrimaryAxis><DefinedDirection>+X</DefinedDirection><Source>ReferenceFrame</Source><SourceDirection>-Z</SourceDirection><FeatureName></FeatureName></PrimaryAxis><SecondaryAxis><DefinedDirection>+Y</DefinedDirection><Source>ReferenceFrame</Source><SourceDirection>+Y</SourceDirection><FeatureName></FeatureName></SecondaryAxis></Value></Frame><Frame><Id>Frame2</Id><Value><Name>F1</Name><Origin><Source>GeometricFeature</Source><FeatureName>cylindrical surface 1</FeatureName></Origin><PrimaryAxis><DefinedDirection>-X</DefinedDirection><Source>ReferenceFrame</Source><SourceDirection>+Z</SourceDirection><FeatureName></FeatureName></PrimaryAxis><SecondaryAxis><DefinedDirection>+Y</DefinedDirection><Source>ReferenceFrame</Source><SourceDirection>+Y</SourceDirection><FeatureName></FeatureName></SecondaryAxis></Value></Frame><Frame><Id>Frame3</Id><Value><Name>Bc1</Name><Origin><Source>GeometricFeature</Source><FeatureName>cylindrical surface 1</FeatureName></Origin><PrimaryAxis><DefinedDirection>+X</DefinedDirection><Source>GeometricFeature</Source><SourceDirection>+Z</SourceDirection><FeatureName>segment 135</FeatureName></PrimaryAxis><SecondaryAxis><DefinedDirection>+Y</DefinedDirection><Source>ReferenceFrame</Source><SourceDirection>+Z</SourceDirection><FeatureName></FeatureName></SecondaryAxis></Value></Frame><Frame><Id>Frame4</Id><Value><Name>BMp</Name><Origin><Source>GeometricFeature</Source><FeatureName>planar surface 11</FeatureName></Origin><PrimaryAxis><DefinedDirection>+X</DefinedDirection><Source>ReferenceFrame</Source><SourceDirection>-Z</SourceDirection><FeatureName></FeatureName></PrimaryAxis><SecondaryAxis><DefinedDirection>+Z</DefinedDirection><Source>ReferenceFrame</Source><SourceDirection>+Y</SourceDirection><FeatureName></FeatureName></SecondaryAxis></Value></Frame></Frames>  GraphicType=FromGeometry  MarkerShape=Sphere  MarkerSize=10  GraphicVisPropType=SimpleVisualProperties  GraphicDiffuseColor=[134 134 71]/255  GraphicSpecularColor=[0.5 0.5 0.5 1.0]  GraphicAmbientColor=[0.15 0.15 0.15 1.0]  GraphicEmissiveColor=[0.0 0.0 0.0 1.0]  GraphicShininess=75  GraphicOpacity=1.0
  Sim-PS1 : nesl_utility/Simulink-PS Converter  PhysicalDomain=network_engine_domain  SubClassName=ps_input  LeftPortType=input  RightPortType=output  PseudoPeriodic=off  Frequencies=[]  NoiseDistribution=none  NoiseParameters=[]  Unit=rad  AffineConversion=off  FilteringAndDerivatives=provide  SimscapeFilterOrder=2  InputFilterTimeConstant=0.001  UdotUserProvided=2
      settings: SourceProductBaseCode=PW,SS
  Sine Wave : Sin  Amplitude=Th1A*Th1f  Frequency=Th1f  Phase=pi/2  SampleTime=0
  Sine Wave1 : Sin  Amplitude=Th1A*Th1f*Th1f  Frequency=Th1f  Phase=pi  SampleTime=0
  Theta1-rotation : sm_lib/Joints/Revolute Joint  JointMode=Normal  SenseConstraintForce=off  SenseConstraintForceX=off  SenseConstraintForceY=off  SenseConstraintForceZ=off  SenseConstraintTorque=off  SenseConstraintTorqueX=off  SenseConstraintTorqueY=off  SenseConstraintTorqueZ=off  SenseTotalForce=off  SenseTotalForceX=off  SenseTotalForceY=off  SenseTotalForceZ=off  SenseTotalTorque=off  SenseTotalTorqueX=off  SenseTotalTorqueY=off  SenseTotalTorqueZ=off  CompositeWrenchDir=FollowerOnBase  CompositeWrenchFrame=BaseFrame  EquilibriumPosition=0  EquilibriumPositionUnits=rad  SpringStiffness=0  SpringStiffnessUnits=N*m/rad  DampingCoefficient=10  DampingCoefficientUnits=N*m/(rad/s)  TorqueActuationMode=NoTorque  MotionActuationMode=InputMotion  SensePosition=off  SenseVelocity=off  SenseAcceleration=off  SenseTorqueForce=off  SenseLowerLimitTorqueForce=off  SenseUpperLimitTorqueForce=off  LowerLimitSpecify=off  LowerLimitBound=-90  LowerLimitBoundUnits=deg  LowerLimitStiffness=1e4  LowerLimitStiffnessUnits=N*m/deg  LowerLimitDamping=10  LowerLimitDampingUnits=N*m/(deg/s)  LowerLimitTransitionRegionWidth=0.1  LowerLimitTransitionRegionWidthUnits=deg  UpperLimitSpecify=off  UpperLimitBound=90  UpperLimitBoundUnits=deg  UpperLimitStiffness=1e4  UpperLimitStiffnessUnits=N*m/deg  UpperLimitDamping=10  UpperLimitDampingUnits=N*m/(deg/s)  UpperLimitTransitionRegionWidth=0.1  UpperLimitTransitionRegionWidthUnits=deg  PositionTargetSpecify=on  PositionTargetPriority=Low  PositionTargetValue=Th1B  PositionTargetValueUnits=rad  VelocityTargetSpecify=off  VelocityTargetPriority=High  VelocityTargetValue=0  VelocityTargetValueUnits=deg/s
  BMp : PMIOPort  Side=Left
  Bc1 : PMIOPort  Port=2  Side=Left
  F1 : PMIOPort  Port=3  Side=Right
  F2_rot : PMIOPort  Port=4  Side=Right
  wires:
  Sine Wave/1 -> Sim-PS1/2
  Sine Wave1/1 -> Sim-PS1/3
  Theta1[rad]/1 -> Sim-PS1/1  "Theta1"
  connections:
  BaseSolid/RConn2 -- BMp/RConn1
  Theta1-rotation/LConn1 -- BaseSolid/LConn1
  Sim-PS1/RConn1 -- Theta1-rotation/LConn2
  F2_rot/RConn1 -- Theta1-rotation/RConn1
  F1/RConn1 -- BaseSolid/RConn1
  Bc1/RConn1 -- BaseSolid/LConn2

== system WMMSupportingForcesGP2020a/Mobile Manipulator in Simscape/Hydraulic manipulator, Simscape/EndMassObject ==
  EndObjectMass : sm_lib/Body Elements/File Solid  ExtGeomFileName=10_ObjectGP.STEP  UnitType=FromFile  ExtGeomFileUnits=m  StepReaderType=OCC  ExportConvexHullGeometry=off  InertiaType=Custom  Mass=570.18877059  MassUnits=kg  CenterOfMass=[2.16142487 0.01347152 0.06601658]  CenterOfMassUnits=m  MomentsOfInertia=[46.81220713 72.19317437 67.11012925]  MomentsOfInertiaUnits=kg*m^2  ProductsOfInertia=[0.04641137 0.08825278 0.37588204]  ProductsOfInertiaUnits=kg*m^2  BasedOnType=Density  Density=7850  DensityUnits=kg/m^3  DoExposeReferenceFrame=off  SerializedFrames=<Frames><Frame><Id>Frame1</Id><Value><Name>P32p</Name><Origin><Source>GeometricFeature</Source><FeatureName>circular curve 7</FeatureName></Origin><PrimaryAxis><DefinedDirection>+Y</DefinedDirection><Source>GeometricFeature</Source><SourceDirection>+Z</SourceDirection><FeatureName>segment 159</FeatureName></PrimaryAxis><SecondaryAxis><DefinedDirection>+X</DefinedDirection><Source>ReferenceFrame</Source><SourceDirection>+X</SourceDirection><FeatureName></FeatureName></SecondaryAxis></Value></Frame><Frame><Id>Frame2</Id><Value><Name>D22</Name><Origin><Source>GeometricFeature</Source><FeatureName>planar surface 154</FeatureName></Origin><PrimaryAxis><DefinedDirection>+Z</DefinedDirection><Source>ReferenceFrame</Source><SourceDirection>+Z</SourceDirection><FeatureName></FeatureName></PrimaryAxis><SecondaryAxis><DefinedDirection>+X</DefinedDirection><Source>ReferenceFrame</Source><SourceDirection>+X</SourceDirection><FeatureName></FeatureName></SecondaryAxis></Value></Frame></Frames>  GraphicType=FromGeometry  MarkerShape=Sphere  MarkerSize=10  GraphicVisPropType=SimpleVisualProperties  GraphicDiffuseColor=[255 9 134]/255  GraphicSpecularColor=[0.5 0.5 0.5 1.0]  GraphicAmbientColor=[0.15 0.15 0.15 1.0]  GraphicEmissiveColor=[0.0 0.0 0.0 1.0]  GraphicShininess=75  GraphicOpacity=1.0
  P32p_to_P32 : sm_lib/Frames and Transforms/Rigid Transform  TranslationMethod=StandardAxis  TranslationStandardOffset=17  TranslationLengthUnit=mm  TranslationStandardAxis=+Z  TranslationCartesianOffset=[0 0 0]  TranslationROffset=0  TranslationROffsetUnits=m  TranslationZOffset=0  TranslationZOffsetUnits=m  TranslationThetaOffset=0  TranslationThetaOffsetUnits=deg  RotationMethod=None  RotationAngleUnits=deg  RotationStandardAxis=+Y  RotationAngle=-90  RotationArbitraryAxis=[0 0 1]  FollAlignAxisA=+X  BaseAlignAxisA=+Y  FollAlignAxisB=+Y  BaseAlignAxisB=+Z  RotationSequenceAxes=FollowerAxes  RotationSequence=XYX  RotationSequenceAngles=[0 0 0]  RotationSequenceAnglesUnits=deg  RotationMatrix=[1 0 0; 0 1 0; 0 0 1]
  P32 : PMIOPort  Side=Left
  D22 : PMIOPort  Port=2  Side=Left
  connections:
  EndObjectMass/LConn1 -- P32p_to_P32/LConn1
  P32p_to_P32/RConn1 -- P32/RConn1
  D22/RConn1 -- EndObjectMass/RConn1
